simulink library "Lib_Turbo_Shaft_TMATS_org"  (Simulink 10.0)
settings: Solver=ode45  StartTime=0.0  StopTime=10.0  RelTol=1e-3  EnableMultiTasking=on
Description:
  | Thomas Modules
settings Model: Creator=jwchapm2  LastModifiedBy=bhisma

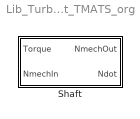
== system Lib_Turbo_Shaft_TMATS_org ==
  Shaft : Subsystem  mask(T-MATS: Shaft Library Block){Shaft_Inertia_M=0.3183}
      mask prompts: Shaft_Inertia_M "Shaft_Inertia_M - Shaft Inertia Term [slugs*ft2]"
      mask help: This block simulates the performance of a shaft using basic dynamic equations and properties.
      mask Help: web(which('Turbo_TMATS_Shft.html'),'-helpbrowser')

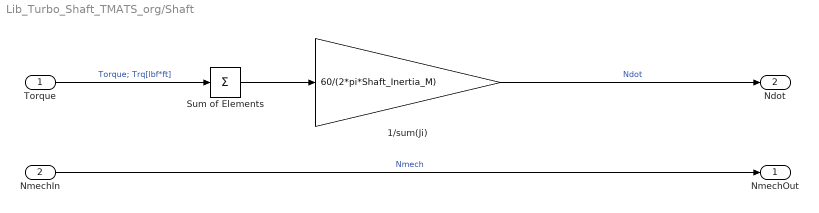
== system Lib_Turbo_Shaft_TMATS_org/Shaft ==
  Torque : Inport
  NmechIn : Inport  Port=2
  1/sum(Ji) : Gain  Gain=60/(2*pi*Shaft_Inertia_M)  SaturateOnIntegerOverflow=on  OutDataTypeStr=Inherit: Same as input  ParamDataTypeStr=Inherit: Same as input
  Sum of Elements : Sum  Inputs=+
  NmechOut : Outport
  Ndot : Outport  Port=2
  wires:
  NmechIn/1 -> NmechOut/1  "Nmech"
  1/sum(Ji)/1 -> Ndot/1  "Ndot"
  Torque/1 -> Sum of Elements/1  "Torque; Trq[lbf*ft]"
  Sum of Elements/1 -> 1/sum(Ji)/1
